simulink model "Lab03_Q1_Sim"  (R2024a)
settings: Solver=VariableStepAuto  StartTime=0.0  StopTime=50  RelTol=1e-3
values from neighbouring files (symbols this model uses):
  C_T = H'    [Lab03_Q1.m]    (also in Lab03_Q1_Data.mat = [0 1])
  G_T = G'    [Lab03_Q1.m]    (also in Lab03_Q1_Data.mat = [0  -0.289176820335; 1  1.26502539796])
  H_T = C'    [Lab03_Q1.m]    (also in Lab03_Q1_Data.mat = [0.0385501764157 0.0229662791138])
  L_db = acker(G_T, H_T, desired_poles_db)    [Lab03_Q1.m]    (also in Lab03_Q1_Data.mat = [20.085372175 21.367447239])
  L_ndb = acker(G_T, H_T, desired_poles_ndb)    [Lab03_Q1.m]    (also in Lab03_Q1_Data.mat = [-1.07836626508 0.287230146767])
settings Model: Creator=24246  LastModifiedBy=24246
settings DataIOCC: InspectSignalLogs=on  ReturnWorkspaceOutputs=off  LoggingFileName=NDB_yk.mat

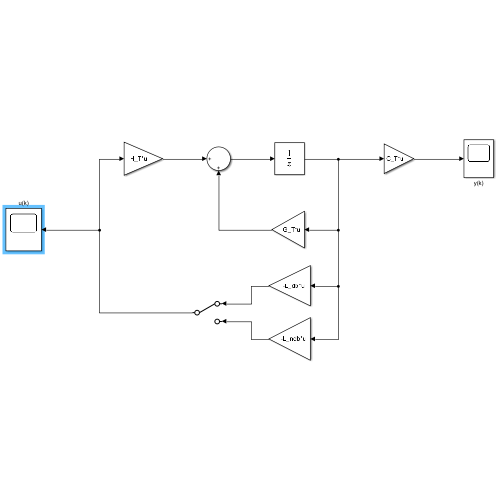
[thumbnail: Simulink's stored preview of the top-level diagram]
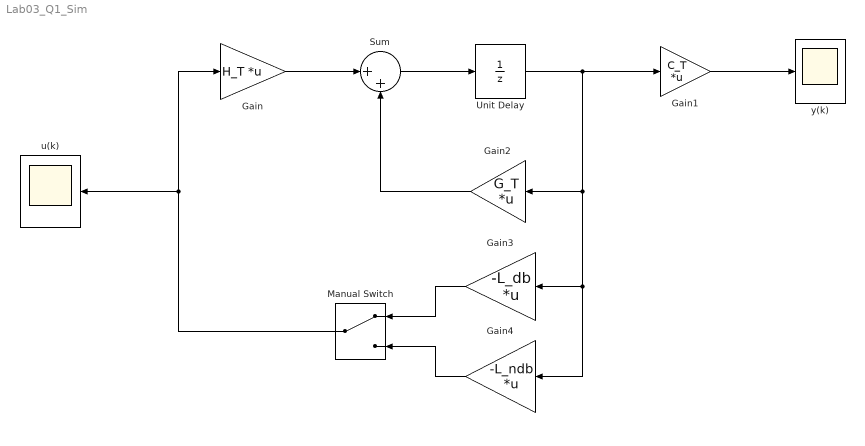
== system Lab03_Q1_Sim ==
  Gain : Gain  Gain=H_T  Multiplication=Matrix(K*u)
  Gain1 : Gain  Gain=C_T  Multiplication=Matrix(K*u)
  Gain2 : Gain  Gain=G_T  Multiplication=Matrix(K*u)
  Gain3 : Gain  Gain=-L_db  Multiplication=Matrix(K*u)
  Gain4 : Gain  Gain=-L_ndb  Multiplication=Matrix(K*u)
  Manual Switch : ManualSwitch
  Sum : Sum  Inputs=|++
  Unit Delay : UnitDelay  InitialCondition=[0 0.3]  SampleTime=-1  HasFrameUpgradeWarning=on
  u(k) : Scope
  y(k) : Scope
  wires:
  Gain/1 -> Sum/1
  Unit Delay/1 -> Gain3/1, Gain4/1, Gain2/1, Gain1/1
  Sum/1 -> Unit Delay/1
  Gain2/1 -> Sum/2
  Gain3/1 -> Manual Switch/1
  Gain4/1 -> Manual Switch/2
  Manual Switch/1 -> Gain/1, u(k)/1
  Gain1/1 -> y(k)/1
